simulink model "simulink_inline_export"  (Simulink 7.9)
settings: Solver=ode45  StartTime=0.0  StopTime=10.0  RelTol=1e-3
undefined symbols (not defined in the file or in its folder): MAX_LIFT, SLIDER_POS
settings Model: Creator=boakes  LastModifiedBy=boakes

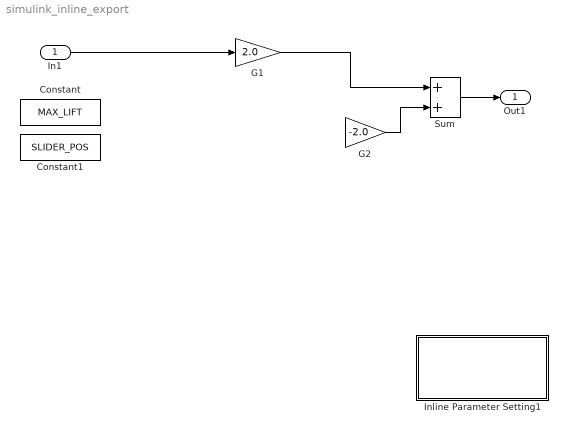
== system simulink_inline_export ==
  In1 : Inport
  Constant : Constant  Value=MAX_LIFT
  Constant1 : Constant  Value=SLIDER_POS
  G1 : Gain  Gain=2.0
  G2 : Gain  Gain=-2.0
  Inline Parameter Setting1 : Subsystem
  Sum : Sum
  Out1 : Outport
  wires:
  G1/1 -> Sum/1
  Sum/1 -> Out1/1
  In1/1 -> G1/1
  G2/1 -> Sum/2

== system simulink_inline_export/Inline Parameter Setting1 ==
